simulink model "eVTOL_System"  (R2024b)
settings: Solver=FixedStepAuto  StartTime=0.0  StopTime=inf  RelTol=1e-3
undefined symbols (not defined in the file): airspeed, Battery, BCE12, BCE_Set_init, BMS_Controller_State, C, Cell10_P, Cell11_P, Cell12_P, Cell13_P, Cell14_P, Cell15_P, Cell16_P, Cell17_P, Cell18_P, Cell19_P, Cell1_N, Cell1_P, Cell20_P, Cell21_P, Cell22_P, Cell23_P, Cell24_P, Cell2_P, Cell3_P, Cell4_P, Cell5_P, Cell6_P, Cell7_P, Cell8_P, Cell9_P, Charging_State, CityMission, control, controlParams, ControlSampleTime, CriticalTiltAngle, currentFactor, CV_Gain, ddx, ddy, ddz, Device_01, Device_02, DiscIntNeverNeededParam, dx, dy, dz, Earth, env, F, F28379D_ADC_MaxCount, F28379D_ADC_Vmax, FixedWingMission, flightState, Foc_Ki_IxTcpu, Foc_Ki_S, Foc_Kp_I, Foc_Kp_S, fractalcoef ... (+68)
libraries: fl_lib x1115, nesl_utility x617, slrealtimeethercatlib x217, simulink x130, canmsglib x101, speedgoatlib_IO611_obsolete x91, slpidlib x49, mcbcontrolslib x44, slrealtimeutilitieslib x35, speedgoatlib_hdlCoder_IO3xx x31, dspstat3 x24, mcbpositiondecoderlib x12
(part 10 of 31)

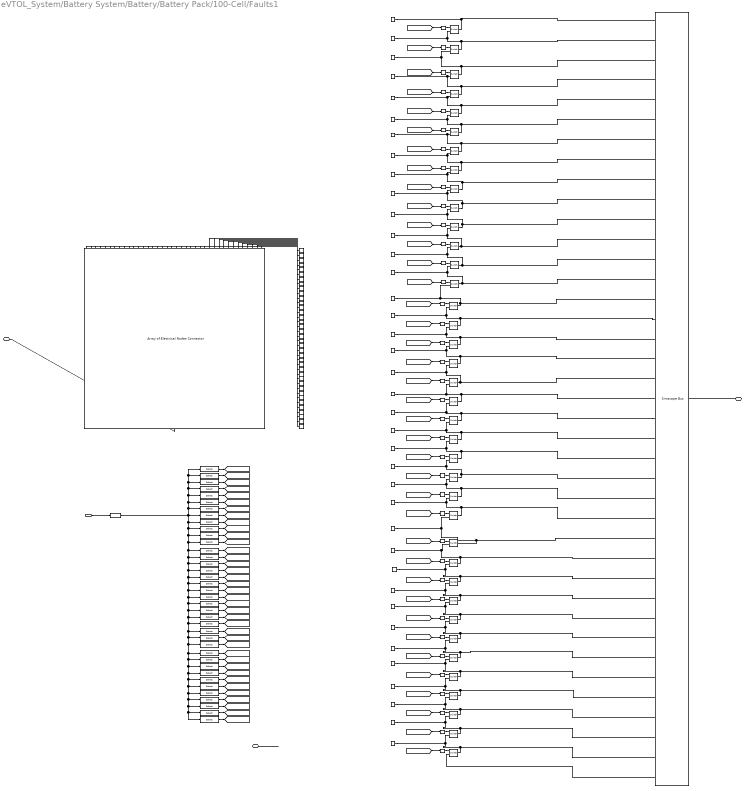
== system eVTOL_System/Battery System/Battery/Battery Pack/100-Cell/Faults1 ==
  note: Short-Circuits
  note: Short-Circuits
  note: Short-Circuits
  Short_Circuits : Inport
  Array of Electrical Nodes Connector : batt_lib/Connectors/Array of Electrical Nodes Connector  numInputConnections=simscape.battery.enum.thermal.numArrayOfNodesConnections.thirtyeight  inNode1NumElements=1  inNode2NumElements=1  inNode3NumElements=1  inNode4NumElements=1  inNode5NumElements=1  inNode6NumElements=1  inNode7NumElements=1  inNode8NumElements=1  inNode9NumElements=1  inNode10NumElements=1  inNode11NumElements=1  inNode12NumElements=1  inNode13NumElements=1  inNode14NumElements=1  inNode15NumElements=1  inNode16NumElements=1  inNode17NumElements=1  inNode18NumElements=1  inNode19NumElements=1  inNode20NumElements=1  inNode21NumElements=1  inNode22NumElements=1  inNode23NumElements=1  inNode24NumElements=1  inNode25NumElements=1  inNode26NumElements=1  inNode27NumElements=1  inNode28NumElements=1  inNode29NumElements=1  inNode30NumElements=1  inNode31NumElements=1  inNode32NumElements=1  inNode33NumElements=1  inNode34NumElements=1  inNode35NumElements=1  inNode36NumElements=1  inNode37NumElements=1  inNode38NumElements=1  inNode39NumElements=1  inNode40NumElements=1  inNode41NumElements=1  inNode42NumElements=1  inNode43NumElements=1  inNode44NumElements=1  inNode45NumElements=1  inNode46NumElements=1  inNode47NumElements=1  inNode48NumElements=1  inNode49NumElements=1  inNode50NumElements=1
      settings: InternalSimscapePortConfiguration="{\"Bottom\":[{\"id\":\"outConn\",\"label\":\"outConn\",\"type\":\"foundation.electrical.electrical\"}],\"Left\":[],\"Right\":[],\"Top\":[{\"id\":\"inConn1\",\"label\":\"inConn1\",\"type\":\"foundation.electrical.electrical\"},{\"id\":\"inConn2\",\"label\":\"inConn2\",\"type\":\"foundation.electrical.electrical\"},{\"id\":\"inConn3\",\"label\":\"inConn3\",\"type\":\"foundation.electrical.electrical\"},{\"id\":\"inConn4\",\"label\":\"inConn4\",\"type\":\"foundation.electrical.electrical\"},{\"id\":\"inConn5\",\"label\":\"inConn5\",\"type\":\"foundation.electrical.electrical\"},{\"id\":\"inConn6\",\"label\":\"inConn6\",\"type\":\"foundation.electrical.electrical\"},{\"id\":\"inConn7\",\"label\":\"inConn7\",\"type\":\"foundation.electrical.electrical\"},{\"id\":\"inConn8\",\"label\":\"inConn8\",\"type\":\"foundation.electrical.electrical\"},{\"id\":\"inConn9\",\"label\":\"inConn9\",\"type\":\"foundation.electrical.electrical\"},{\"id\":\"inConn10\",\"label\":\"inConn10\",\"type\":\"foundation.electrical.electrical\"},{\"id\":\"inConn11\",\"label\":\"inConn11\",\"type\":\"foundation.electrical.electrical\"},{\"id\":\"inConn12\",\"label\":\"inConn12\",\"type\":\"foundation.electrical.electrical\"},{\"id\":\"inConn13\",\"label\":\"inConn13\",\"type\":\"foundation.electrical.electrical\"},{\"id\":\"inConn14\",\"label\":\"inConn14\",\"type\":\"foundation.electrical.electrical\"},{\"id\":\"inConn15\",\"label\":\"inConn15\",\"type\":\"foundation.electrical.electrical\"},{\"id\":\"inConn16\",\"label\":\"inConn16\",\"type\":\"foundation.electrical.electrical\"},{\"id\":\"inConn17\",\"label\":\"inConn17\",\"type\":\"foundation.electrical.electrical\"},{\"id\":\"inConn18\",\"label\":\"inConn18\",\"type\":\"foundation.electrical.electrical\"},{\"id\":\"inConn19\",\"label\":\"inConn19\",\"type\":\"foundation.electrical.electrical\"},{\"id\":\"inConn20\",\"label\":\"inConn20\",\"type\":\"foundation.electrical.electrical\"},{\"id\":\"inConn21\",\"label\":\"inConn21\",\"type\":\"foundation.electrical.electrical\"},{\"id\":\"inConn22\",\"label\":\"inConn22\",\"type\":\"foundation.electrical.electrical\"},{\"id\":\"inConn23\",\"label\":\"inConn23\",\"type\":\"foundation.electrical.electrical\"},{\"id\":\"inConn24\",\"label\":\"inConn24\",\"type\":\"foundation.electrical.electrical\"},{\"id\":\"inConn25\",\"label\":\"inConn25\",\"type\":\"foundation.electrical.electrical\"},{\"id\":\"inConn26\",\"label\":\"inConn26\",\"type\":\"foundation.electrical.electrical\"},{\"id\":\"inConn27\",\"label\":\"inConn27\",\"type\":\"foundation.electrical.electrical\"},{\"id\":\"inConn28\",\"label\":\"inConn28\",\"type\":\"foundation.electrical.electrical\"},{\"id\":\"inConn29\",\"label\":\"inConn29\",\"type\":\"foundation.electrical.electrical\"},{\"id\":\"inConn30\",\"label\":\"inConn30\",\"type\":\"foundation.electrical.electrical\"},{\"id\":\"inConn31\",\"label\":\"inConn31\",\"type\":\"foundation.electrical.electrical\"},{\"id\":\"inConn32\",\"label\":\"inConn32\",\"type\":\"foundation.electrical.electrical\"},{\"id\":\"inConn33\",\"label\":\"inConn33\",\"type\":\"foundation.electrical.electrical\"},{\"id\":\"inConn34\",\"label\":\"inConn34\",\"type\":\"foundation.electrical.electrical\"},{\"id\":\"inConn35\",\"label\":\"inConn35\",\"type\":\"foundation.electrical.electrical\"},{\"id\":\"inConn36\",\"label\":\"inConn36\",\"type\":\"foundation.electrical.electrical\"},{\"id\":\"inConn37\",\"label\":\"inConn37\",\"type\":\"foundation.electrical.electrical\"},{\"id\":\"inConn38\",\"label\":\"inConn38\",\"type\":\"foundation.electrical.electrical\"}]}"
  Connection Label : ConnectionLabel  Label=pos1
  Connection Label1 : ConnectionLabel  Label=pos7
  Connection Label10 : ConnectionLabel  Label=pos3
  Connection Label100 : ConnectionLabel  Label=pos12
  Connection Label101 : ConnectionLabel  Label=pos11
  Connection Label102 : ConnectionLabel  Label=pos10
  Connection Label103 : ConnectionLabel  Label=pos9
  Connection Label104 : ConnectionLabel  Label=pos8
  Connection Label105 : ConnectionLabel  Label=pos7
  Connection Label106 : ConnectionLabel  Label=pos6
  Connection Label107 : ConnectionLabel  Label=pos5
  Connection Label108 : ConnectionLabel  Label=pos4
  Connection Label109 : ConnectionLabel  Label=pos3
  Connection Label11 : ConnectionLabel  Label=pos2
  Connection Label110 : ConnectionLabel  Label=pos2
  Connection Label111 : ConnectionLabel  Label=pos1
  Connection Label112 : ConnectionLabel  Label=pos24
  Connection Label113 : ConnectionLabel  Label=pos23
  Connection Label114 : ConnectionLabel  Label=pos22
  Connection Label115 : ConnectionLabel  Label=pos21
  Connection Label116 : ConnectionLabel  Label=pos20
  Connection Label117 : ConnectionLabel  Label=pos19
  Connection Label118 : ConnectionLabel  Label=pos18
  Connection Label119 : ConnectionLabel  Label=pos17
  Connection Label12 : ConnectionLabel  Label=pos29
  Connection Label120 : ConnectionLabel  Label=pos16
  Connection Label121 : ConnectionLabel  Label=pos15
  Connection Label122 : ConnectionLabel  Label=pos14
  Connection Label123 : ConnectionLabel  Label=pos13
  Connection Label13 : ConnectionLabel  Label=pos28
  Connection Label14 : ConnectionLabel  Label=pos27
  Connection Label15 : ConnectionLabel  Label=pos26
  Connection Label16 : ConnectionLabel  Label=pos25
  Connection Label17 : ConnectionLabel  Label=pos34
  Connection Label18 : ConnectionLabel  Label=pos33
  Connection Label19 : ConnectionLabel  Label=pos32
  Connection Label2 : ConnectionLabel  Label=pos8
  Connection Label20 : ConnectionLabel  Label=pos31
  Connection Label21 : ConnectionLabel  Label=pos30
  Connection Label23 : ConnectionLabel  Label=pos38
  Connection Label3 : ConnectionLabel  Label=pos9
  Connection Label4 : ConnectionLabel  Label=pos10
  Connection Label45 : ConnectionLabel  Label=pos37
  Connection Label48 : ConnectionLabel  Label=pos36
  Connection Label49 : ConnectionLabel  Label=pos35
  Connection Label5 : ConnectionLabel  Label=pos11
  Connection Label6 : ConnectionLabel  Label=pos12
  Connection Label7 : ConnectionLabel  Label=pos6
  Connection Label74 : ConnectionLabel  Label=pos13
  Connection Label75 : ConnectionLabel  Label=pos19
  Connection Label76 : ConnectionLabel  Label=pos15
  Connection Label77 : ConnectionLabel  Label=pos14
  Connection Label78 : ConnectionLabel  Label=pos20
  Connection Label79 : ConnectionLabel  Label=pos21
  Connection Label8 : ConnectionLabel  Label=pos5
  Connection Label80 : ConnectionLabel  Label=pos22
  Connection Label81 : ConnectionLabel  Label=pos23
  Connection Label82 : ConnectionLabel  Label=pos24
  Connection Label83 : ConnectionLabel  Label=pos18
  Connection Label84 : ConnectionLabel  Label=pos17
  Connection Label85 : ConnectionLabel  Label=pos16
  Connection Label86 : ConnectionLabel  Label=pos25
  Connection Label87 : ConnectionLabel  Label=pos31
  Connection Label88 : ConnectionLabel  Label=pos27
  Connection Label89 : ConnectionLabel  Label=pos26
  Connection Label9 : ConnectionLabel  Label=pos4
  Connection Label90 : ConnectionLabel  Label=pos32
  Connection Label91 : ConnectionLabel  Label=pos33
  Connection Label92 : ConnectionLabel  Label=pos34
  Connection Label93 : ConnectionLabel  Label=pos35
  Connection Label94 : ConnectionLabel  Label=pos36
  Connection Label95 : ConnectionLabel  Label=pos30
  Connection Label96 : ConnectionLabel  Label=pos29
  Connection Label97 : ConnectionLabel  Label=pos28
  Connection Label98 : ConnectionLabel  Label=pos37
  Connection Label99 : ConnectionLabel  Label=pos38
  Data Type Conversion1 : DataTypeConversion  OutDataTypeStr=double  SaturateOnIntegerOverflow=off  RndMeth=Floor
  Selector1 : Selector  IndexOptions=Index vector (dialog)  Indices=35  OutputSizes=1
  Selector10 : Selector  IndexOptions=Index vector (dialog)  Indices=25  OutputSizes=1
  Selector11 : Selector  IndexOptions=Index vector (dialog)  Indices=26  OutputSizes=1
  Selector12 : Selector  IndexOptions=Index vector (dialog)  Indices=28  OutputSizes=1
  Selector13 : Selector  IndexOptions=Index vector (dialog)  Indices=38  OutputSizes=1
  Selector14 : Selector  IndexOptions=Index vector (dialog)  Indices=48  OutputSizes=1
  Selector15 : Selector  IndexOptions=Index vector (dialog)  Indices=47  OutputSizes=1
  Selector16 : Selector  IndexOptions=Index vector (dialog)  Indices=45  OutputSizes=1
  Selector17 : Selector  IndexOptions=Index vector (dialog)  Indices=40  OutputSizes=1
  Selector18 : Selector  IndexOptions=Index vector (dialog)  Indices=39  OutputSizes=1
  Selector19 : Selector  IndexOptions=Index vector (dialog)  Indices=42  OutputSizes=1
  Selector2 : Selector  IndexOptions=Index vector (dialog)  Indices=33  OutputSizes=1
  Selector20 : Selector  IndexOptions=Index vector (dialog)  Indices=44  OutputSizes=1
  Selector21 : Selector  IndexOptions=Index vector (dialog)  Indices=37  OutputSizes=1
  Selector22 : Selector  IndexOptions=Index vector (dialog)  Indices=43  OutputSizes=1
  Selector23 : Selector  IndexOptions=Index vector (dialog)  Indices=41  OutputSizes=1
  Selector24 : Selector  IndexOptions=Index vector (dialog)  Indices=46  OutputSizes=1
  Selector25 : Selector  IndexOptions=Index vector (dialog)  Indices=51  OutputSizes=1
  Selector26 : Selector  IndexOptions=Index vector (dialog)  Indices=50  OutputSizes=1
  Selector27 : Selector  IndexOptions=Index vector (dialog)  Indices=53  OutputSizes=1
  Selector29 : Selector  IndexOptions=Index vector (dialog)  Indices=62  OutputSizes=1
  Selector3 : Selector  IndexOptions=Index vector (dialog)  Indices=34  OutputSizes=1
  Selector30 : Selector  IndexOptions=Index vector (dialog)  Indices=60  OutputSizes=1
  Selector31 : Selector  IndexOptions=Index vector (dialog)  Indices=55  OutputSizes=1
  Selector32 : Selector  IndexOptions=Index vector (dialog)  Indices=54  OutputSizes=1
  Selector33 : Selector  IndexOptions=Index vector (dialog)  Indices=57  OutputSizes=1
  Selector34 : Selector  IndexOptions=Index vector (dialog)  Indices=59  OutputSizes=1
  Selector35 : Selector  IndexOptions=Index vector (dialog)  Indices=52  OutputSizes=1
  Selector36 : Selector  IndexOptions=Index vector (dialog)  Indices=58  OutputSizes=1
  Selector37 : Selector  IndexOptions=Index vector (dialog)  Indices=56  OutputSizes=1
  Selector38 : Selector  IndexOptions=Index vector (dialog)  Indices=61  OutputSizes=1
  Selector39 : Selector  IndexOptions=Index vector (dialog)  Indices=49  OutputSizes=1
  Selector4 : Selector  IndexOptions=Index vector (dialog)  Indices=31  OutputSizes=1
  Selector5 : Selector  IndexOptions=Index vector (dialog)  Indices=29  OutputSizes=1
  Selector6 : Selector  IndexOptions=Index vector (dialog)  Indices=36  OutputSizes=1
  Selector7 : Selector  IndexOptions=Index vector (dialog)  Indices=30  OutputSizes=1
  Selector8 : Selector  IndexOptions=Index vector (dialog)  Indices=32  OutputSizes=1
  Selector9 : Selector  IndexOptions=Index vector (dialog)  Indices=27  OutputSizes=1
  Simscape Bus : SimscapeBus  HierarchyStrings=Cell38_P;Cell37_P;Cell36_P;Cell35_P;Cell34_P;Cell33_P;Cell32_P;Cell31_P;Cell30_P;Cell29_P;Cell28_P;Cell27_P;Cell26_P;Cell25_P;Cell24_P;Cell23_P;Cell22_P;Cell21_P;Cell20_P;Cell19_P;Cell18_P;Cell17_P;Cell16_P;Cell15_P;Cell14_P;Cell13_P;Cell12_P;Cell11_P;Cell10_P;Cell9_P;Cell8_P;Cell7_P;Cell6_P;Cell5_P;Cell4_P;Cell3_P;Cell2_P;Cell1_P;Cell1_N
  Simulink-PS Converter{1..38} (38 alike) : nesl_utility/Simulink-PS Converter  PhysicalDomain=network_engine_domain  SubClassName=ps_input  LeftPortType=input  RightPortType=output  PseudoPeriodic=off  Frequencies=[]  NoiseDistribution=none  NoiseParameters=[]  Unit=1  AffineConversion=off  FilteringAndDerivatives=zero  SimscapeFilterOrder=1  InputFilterTimeConstant=0.001  UdotUserProvided=1
  Switch{,1..37} (38 alike) : fl_lib/Electrical/Electrical Elements/Switch  R_closed=0.01 Ohm  G_open=1e-8 1/Ohm  Threshold=0.5  i_specify=off  i_priority=None  i=0 A  i_nominal_specify=off  i_nominal_value=1  i_nominal_unit=A  v_specify=off  v_priority=None  v=0 V  v_nominal_specify=off  v_nominal_value=1  v_nominal_unit=V
  +Bus : PMIOPort  Side=Right
  Cells : PMIOPort  Port=2  Side=Right
  =Bus : PMIOPort  Port=3  Side=Right
  wires:
  [Cell37_Switch_SC] -> Simulink-PS Converter24/1
  [Cell36_Switch_SC] -> Simulink-PS Converter23/1
  [Cell38_Switch_SC] -> Simulink-PS Converter25/1
  [Cell27_Switch_SC] -> Simulink-PS Converter14/1
  [Cell28_Switch_SC] -> Simulink-PS Converter15/1
  [Cell35_Switch_SC] -> Simulink-PS Converter22/1
  [Cell31_Switch_SC] -> Simulink-PS Converter18/1
  [Cell34_Switch_SC] -> Simulink-PS Converter21/1
  [Cell29_Switch_SC] -> Simulink-PS Converter16/1
  [Cell30_Switch_SC] -> Simulink-PS Converter17/1
  [Cell33_Switch_SC] -> Simulink-PS Converter20/1
  [Cell32_Switch_SC] -> Simulink-PS Converter19/1
  Short_Circuits/1 -> Data Type Conversion1/1
  [Cell23_Switch_SC] -> Simulink-PS Converter9/1
  [Cell20_Switch_SC] -> Simulink-PS Converter6/1
  [Cell17_Switch_SC] -> Simulink-PS Converter3/1
  [Cell18_Switch_SC] -> Simulink-PS Converter4/1
  [Cell26_Switch_SC] -> Simulink-PS Converter12/1
  [Cell19_Switch_SC] -> Simulink-PS Converter5/1
  [Cell25_Switch_SC] -> Simulink-PS Converter11/1
  [Cell22_Switch_SC] -> Simulink-PS Converter8/1
  [Cell15_Switch_SC] -> Simulink-PS Converter1/1
  [Cell24_Switch_SC] -> Simulink-PS Converter10/1
  [Cell21_Switch_SC] -> Simulink-PS Converter7/1
  [Cell16_Switch_SC] -> Simulink-PS Converter2/1
  [Cell5_Switch_SC] -> Simulink-PS Converter30/1
  [Cell4_Switch_SC] -> Simulink-PS Converter29/1
  [Cell10_Switch_SC] -> Simulink-PS Converter35/1
  [Cell12_Switch_SC] -> Simulink-PS Converter26/1
  [Cell3_Switch_SC] -> Simulink-PS Converter13/1
  [Cell9_Switch_SC] -> Simulink-PS Converter34/1
  [Cell14_Switch_SC] -> Simulink-PS Converter28/1
  [Cell13_Switch_SC] -> Simulink-PS Converter27/1
  [Cell6_Switch_SC] -> Simulink-PS Converter31/1
  [Cell11_Switch_SC] -> Simulink-PS Converter36/1
  [Cell7_Switch_SC] -> Simulink-PS Converter32/1
  [Cell8_Switch_SC] -> Simulink-PS Converter33/1
  [Cell2_Switch_SC] -> Simulink-PS Converter38/1
  [Cell1_Switch_SC] -> Simulink-PS Converter37/1
  Selector25/1 -> [Cell27_Switch_SC]
  Selector38/1 -> [Cell37_Switch_SC]
  Selector21/1 -> [Cell13_Switch_SC]
  Selector19/1 -> [Cell18_Switch_SC]
  Selector33/1 -> [Cell33_Switch_SC]
  Selector32/1 -> [Cell30_Switch_SC]
  Selector29/1 -> [Cell38_Switch_SC]
  Selector24/1 -> [Cell22_Switch_SC]
  Selector14/1 -> [Cell24_Switch_SC]
  Selector23/1 -> [Cell17_Switch_SC]
  Selector18/1 -> [Cell15_Switch_SC]
  Selector16/1 -> [Cell21_Switch_SC]
  Selector17/1 -> [Cell16_Switch_SC]
  Selector22/1 -> [Cell19_Switch_SC]
  Selector2/1 -> [Cell9_Switch_SC]
  Selector7/1 -> [Cell6_Switch_SC]
  Selector5/1 -> [Cell5_Switch_SC]
  Selector10/1 -> [Cell1_Switch_SC]
  Selector1/1 -> [Cell11_Switch_SC]
  Selector12/1 -> [Cell4_Switch_SC]
  Selector3/1 -> [Cell10_Switch_SC]
  Selector11/1 -> [Cell2_Switch_SC]
  Selector9/1 -> [Cell3_Switch_SC]
  Selector4/1 -> [Cell7_Switch_SC]
  Selector39/1 -> [Cell25_Switch_SC]
  Selector26/1 -> [Cell26_Switch_SC]
  Selector27/1 -> [Cell29_Switch_SC]
  Selector31/1 -> [Cell31_Switch_SC]
  Data Type Conversion1/1 -> Selector4/1, Selector8/1, Selector2/1, Selector3/1, Selector1/1, Selector6/1, Selector7/1, Selector5/1, Selector12/1, Selector9/1, Selector11/1, Selector30/1, Selector29/1, Selector38/1, Selector34/1, Selector36/1, Selector33/1, Selector37/1, Selector31/1, Selector32/1, Selector27/1, Selector35/1, Selector25/1, Selector26/1, Selector39/1, Selector14/1, Selector15/1, Selector24/1, Selector16/1, Selector20/1, Selector22/1, Selector19/1, Selector23/1, Selector17/1, Selector18/1, Selector13/1, Selector21/1, Selector10/1
  Selector13/1 -> [Cell14_Switch_SC]
  Selector30/1 -> [Cell36_Switch_SC]
  Selector15/1 -> [Cell23_Switch_SC]
  Selector36/1 -> [Cell34_Switch_SC]
  Selector20/1 -> [Cell20_Switch_SC]
  Selector8/1 -> [Cell8_Switch_SC]
  Selector34/1 -> [Cell35_Switch_SC]
  Selector37/1 -> [Cell32_Switch_SC]
  Selector35/1 -> [Cell28_Switch_SC]
  Selector6/1 -> [Cell12_Switch_SC]
  connections:
  Simulink-PS Converter17/RConn1 -- Switch3/RConn1
  Switch3/LConn1 -- Connection Label21/LConn1 -- Switch2/RConn2 -- Simscape Bus/LConn30
  Switch6/LConn1 -- Connection Label18/LConn1 -- Switch5/RConn2 -- Simscape Bus/LConn33
  Switch7/LConn1 -- Connection Label17/LConn1 -- Switch6/RConn2 -- Simscape Bus/LConn34
  Switch2/LConn1 -- Switch1/RConn2 -- Connection Label12/LConn1 -- Simscape Bus/LConn29
  Simulink-PS Converter16/RConn1 -- Switch2/RConn1
  Simulink-PS Converter19/RConn1 -- Switch5/RConn1
  Switch10/LConn1 -- Connection Label45/LConn1 -- Switch9/RConn2 -- Simscape Bus/LConn37
  Simulink-PS Converter25/RConn1 -- Switch11/RConn1
  Switch11/LConn1 -- Connection Label23/LConn1 -- Switch10/RConn2 -- Simscape Bus/LConn38
  Switch9/LConn1 -- Switch8/RConn2 -- Connection Label48/LConn1 -- Simscape Bus/LConn36
  Simulink-PS Converter14/RConn1 -- Switch/RConn1
  Simscape Bus/LConn39 -- Switch11/RConn2
  Simulink-PS Converter18/RConn1 -- Switch4/RConn1
  Switch4/LConn1 -- Connection Label20/LConn1 -- Switch3/RConn2 -- Simscape Bus/LConn31
  Simulink-PS Converter24/RConn1 -- Switch10/RConn1
  Switch8/LConn1 -- Switch7/RConn2 -- Connection Label49/LConn1 -- Simscape Bus/LConn35
  Simulink-PS Converter20/RConn1 -- Switch6/RConn1
  Simulink-PS Converter15/RConn1 -- Switch1/RConn1
  Simulink-PS Converter21/RConn1 -- Switch7/RConn1
  Simulink-PS Converter23/RConn1 -- Switch9/RConn1
  Simulink-PS Converter22/RConn1 -- Switch8/RConn1
  Switch5/LConn1 -- Connection Label19/LConn1 -- Switch4/RConn2 -- Simscape Bus/LConn32
  Simscape Bus/LConn27 -- Switch15/RConn2 -- Connection Label14/LConn1 -- Switch/LConn1
  Switch1/LConn1 -- Switch/RConn2 -- Connection Label13/LConn1 -- Simscape Bus/LConn28
  =Bus/RConn1 -- ?
  Array of Electrical Nodes Connector/RConn1 -- +Bus/RConn1
  Switch17/LConn1 -- Simscape Bus/LConn18 -- Connection Label118/LConn1 -- Switch16/RConn2
  Switch14/LConn1 -- Simscape Bus/LConn25 -- Switch23/RConn2 -- Connection Label16/LConn1
  Switch19/LConn1 -- Switch18/RConn2 -- Connection Label116/LConn1 -- Simscape Bus/LConn20
  Switch13/LConn1 -- Simscape Bus/LConn16 -- Connection Label120/LConn1 -- Switch12/RConn2
  Switch22/LConn1 -- Simscape Bus/LConn23 -- Connection Label113/LConn1 -- Switch21/RConn2
  Switch18/LConn1 -- Switch17/RConn2 -- Connection Label117/LConn1 -- Simscape Bus/LConn19
  Switch16/LConn1 -- Simscape Bus/LConn17 -- Connection Label119/LConn1 -- Switch13/RConn2
  Switch27/RConn2 -- Connection Label121/LConn1 -- Switch12/LConn1 -- Simscape Bus/LConn15
  Switch21/LConn1 -- Connection Label114/LConn1 -- Switch20/RConn2 -- Simscape Bus/LConn22
  Simscape Bus/LConn21 -- Switch19/RConn2 -- Connection Label115/LConn1 -- Switch20/LConn1
  Simulink-PS Converter12/RConn1 -- Switch15/RConn1
  Simulink-PS Converter7/RConn1 -- Switch20/RConn1
  Simulink-PS Converter10/RConn1 -- Switch23/RConn1
  Simulink-PS Converter2/RConn1 -- Switch13/RConn1
  Simulink-PS Converter3/RConn1 -- Switch16/RConn1
  Simulink-PS Converter1/RConn1 -- Switch12/RConn1
  Simulink-PS Converter11/RConn1 -- Switch14/RConn1
  Simulink-PS Converter8/RConn1 -- Switch21/RConn1
  Simulink-PS Converter9/RConn1 -- Switch22/RConn1
  Simulink-PS Converter5/RConn1 -- Switch18/RConn1
  Simulink-PS Converter6/RConn1 -- Switch19/RConn1
  Simulink-PS Converter4/RConn1 -- Switch17/RConn1
  Switch15/LConn1 -- Simscape Bus/LConn26 -- Connection Label15/LConn1 -- Switch14/RConn2
  Simscape Bus/LConn24 -- Switch23/LConn1 -- Connection Label112/LConn1 -- Switch22/RConn2
  Cells/RConn1 -- Simscape Bus/RConn1
  Switch33/LConn1 -- Simscape Bus/LConn10 -- Connection Label102/LConn1 -- Switch32/RConn2
  Switch24/LConn1 -- Connection Label109/LConn1 -- Switch37/RConn2 -- Simscape Bus/LConn3
  Switch34/LConn1 -- Connection Label101/LConn1 -- Switch33/RConn2 -- Simscape Bus/LConn11
  Switch25/LConn1 -- Connection Label108/LConn1 -- Switch24/RConn2 -- Simscape Bus/LConn4
  Switch31/LConn1 -- Simscape Bus/LConn8 -- Connection Label104/LConn1 -- Switch30/RConn2
  Switch27/LConn1 -- Switch26/RConn2 -- Connection Label122/LConn1 -- Simscape Bus/LConn14
  Switch26/LConn1 -- Switch35/RConn2 -- Connection Label123/LConn1 -- Simscape Bus/LConn13
  Switch30/LConn1 -- Connection Label105/LConn1 -- Switch29/RConn2 -- Simscape Bus/LConn7
  Switch32/LConn1 -- Connection Label103/LConn1 -- Switch31/RConn2 -- Simscape Bus/LConn9
  Switch29/LConn1 -- Connection Label106/LConn1 -- Switch28/RConn2 -- Simscape Bus/LConn6
  Switch28/LConn1 -- Connection Label107/LConn1 -- Switch25/RConn2 -- Simscape Bus/LConn5
  Switch35/LConn1 -- Connection Label100/LConn1 -- Switch34/RConn2 -- Simscape Bus/LConn12
  Simulink-PS Converter31/RConn1 -- Switch29/RConn1
  Simulink-PS Converter13/RConn1 -- Switch24/RConn1
  Simulink-PS Converter28/RConn1 -- Switch27/RConn1
  Simulink-PS Converter35/RConn1 -- Switch33/RConn1
  Simulink-PS Converter34/RConn1 -- Switch32/RConn1
  Simulink-PS Converter33/RConn1 -- Switch31/RConn1
  Simulink-PS Converter27/RConn1 -- Switch26/RConn1
  Simulink-PS Converter32/RConn1 -- Switch30/RConn1
  Simulink-PS Converter29/RConn1 -- Switch25/RConn1
  Simulink-PS Converter36/RConn1 -- Switch34/RConn1
  Simulink-PS Converter30/RConn1 -- Switch28/RConn1
  Simulink-PS Converter26/RConn1 -- Switch35/RConn1
  Simscape Bus/LConn1 -- Connection Label111/LConn1 -- Switch36/LConn1
  Switch37/LConn1 -- Simscape Bus/LConn2 -- Switch36/RConn2 -- Connection Label110/LConn1
  Simulink-PS Converter37/RConn1 -- Switch36/RConn1
  Simulink-PS Converter38/RConn1 -- Switch37/RConn1
  Connection Label/LConn1 -- Array of Electrical Nodes Connector/LConn1
  Connection Label11/LConn1 -- Array of Electrical Nodes Connector/LConn2
  Connection Label10/LConn1 -- Array of Electrical Nodes Connector/LConn3
  Connection Label9/LConn1 -- Array of Electrical Nodes Connector/LConn4
  Connection Label8/LConn1 -- Array of Electrical Nodes Connector/LConn5
  Connection Label7/LConn1 -- Array of Electrical Nodes Connector/LConn6
  Connection Label1/LConn1 -- Array of Electrical Nodes Connector/LConn7
  Connection Label2/LConn1 -- Array of Electrical Nodes Connector/LConn8
  Connection Label3/LConn1 -- Array of Electrical Nodes Connector/LConn9
  Connection Label4/LConn1 -- Array of Electrical Nodes Connector/LConn10
  Connection Label5/LConn1 -- Array of Electrical Nodes Connector/LConn11
  Connection Label6/LConn1 -- Array of Electrical Nodes Connector/LConn12
  Connection Label74/LConn1 -- Array of Electrical Nodes Connector/LConn13
  Connection Label77/LConn1 -- Array of Electrical Nodes Connector/LConn14
  Connection Label76/LConn1 -- Array of Electrical Nodes Connector/LConn15
  Connection Label85/LConn1 -- Array of Electrical Nodes Connector/LConn16
  Connection Label84/LConn1 -- Array of Electrical Nodes Connector/LConn17
  Connection Label83/LConn1 -- Array of Electrical Nodes Connector/LConn18
  Connection Label75/LConn1 -- Array of Electrical Nodes Connector/LConn19
  Connection Label78/LConn1 -- Array of Electrical Nodes Connector/LConn20
  Connection Label79/LConn1 -- Array of Electrical Nodes Connector/LConn21
  Connection Label80/LConn1 -- Array of Electrical Nodes Connector/LConn22
  Connection Label81/LConn1 -- Array of Electrical Nodes Connector/LConn23
  Connection Label82/LConn1 -- Array of Electrical Nodes Connector/LConn24
  Connection Label86/LConn1 -- Array of Electrical Nodes Connector/LConn25
  Connection Label89/LConn1 -- Array of Electrical Nodes Connector/LConn26
  Connection Label88/LConn1 -- Array of Electrical Nodes Connector/LConn27
  Connection Label97/LConn1 -- Array of Electrical Nodes Connector/LConn28
  Connection Label96/LConn1 -- Array of Electrical Nodes Connector/LConn29
  Connection Label95/LConn1 -- Array of Electrical Nodes Connector/LConn30
  Connection Label87/LConn1 -- Array of Electrical Nodes Connector/LConn31
  Connection Label90/LConn1 -- Array of Electrical Nodes Connector/LConn32
  Connection Label91/LConn1 -- Array of Electrical Nodes Connector/LConn33
  Connection Label92/LConn1 -- Array of Electrical Nodes Connector/LConn34
  Connection Label93/LConn1 -- Array of Electrical Nodes Connector/LConn35
  Connection Label94/LConn1 -- Array of Electrical Nodes Connector/LConn36
  Connection Label98/LConn1 -- Array of Electrical Nodes Connector/LConn37
  Connection Label99/LConn1 -- Array of Electrical Nodes Connector/LConn38
